simulink model "doc_interleaver"  (R2014a)
settings: Solver=ode45  SolverMode=SingleTasking  StartTime=0.0  StopTime=length(errors)  RelTol=1e-3
undefined symbols (not defined in the file or in its folder): gfprimfd
libraries: commblkcod2 x2, commblkintrlv2 x2, commrandsrc2 x1, commsink2 x1, simulink x1, dspsrcs4 x1
settings Model: Creator=The MathWorks Inc.
settings DataIOCC: SignalLoggingSaveFormat=ModelDataLogs  SaveOutput=off  SaveTime=off
settings OptimizationCC: BooleanDataType=off  InlineParams=on  ExpressionDepthLimit=2147483647
settings DebuggingCC: AlgebraicLoopMsg=error  SaveWithParameterizedLinksMsg=none  UnderspecifiedInitializationDetection=Classic  SignalResolutionControl=TryResolveAllWithWarning  SolverPrmCheckMsg=none  MultiTaskDSMMsg=warning  MultiTaskCondExecSysMsg=none  FcnCallInpInsideContextMsg=UseLocalSettings  StateNameClashWarn=warning  StrictBusMsg=None
settings HardwareCC: TargetUnknown=on
settings RTWCC: IncludeERTFirstTime=on
settings GRTTargetCC: CombineOutputUpdateFcns=off  GRTInterface=on

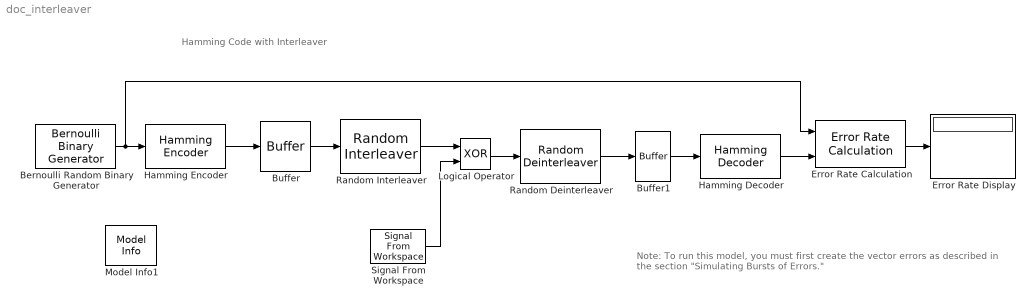
== system doc_interleaver ==
  note: Hamming Code with Interleaver
  note: Note: To run this model, you must first create the vector errors
      | as described in the section "Simulating Bursts of Errors."
  Bernoulli Random Binary Generator : commrandsrc2/Bernoulli Binary Generator  P=0.5  seed=435345  Ts=1  frameBased=on  sampPerFrame=4  orient=off  outDataType=double
  Buffer : Buffer  N=84  TreatMby1Signals=One channel
  Buffer1 : Buffer  N=7  TreatMby1Signals=One channel
  Error Rate Calculation : commsink2/Error Rate Calculation  N=(4/7)*84  st_delay=100  cp_mode=Entire frame  subframe=[]  PMode=Port  WsName=ErrorVec  RsMode2=off  stop=off  numErr=100  maxBits=1000
  Error Rate Display : Display
  Hamming Decoder : commblkcod2/Hamming Decoder  n=7  k=gfprimfd(3,'min')
  Hamming Encoder : commblkcod2/Hamming Encoder  n=7  k=gfprimfd(3,'min')
  Logical Operator : Logic  Operator=XOR
  Model Info1 : simulink/Model-Wide Utilities/Model Info  InitialBlockCM=None  BlockCM=None  Frame=on  DisplayStringWithTags=Info  HorizontalTextAlignment=Center  LeftAlignmentValue=0.5  SourceBlockDiagram=doc_interleaver  TagMaxNumber=20
  Random Deinterleaver : commblkintrlv2/Random Deinterleaver  N=84  seed=113
  Random Interleaver : commblkintrlv2/Random Interleaver  N=84  seed=113
  Signal From Workspace : dspsrcs4/Signal From Workspace  X=errors  Ts=4/7  nsamps=84  OutputAfterFinalValue=Setting to zero  ignoreOrWarnInputAndFrameLengths=off
  wires:
  Error Rate Calculation/1 -> Error Rate Display/1
  Hamming Decoder/1 -> Error Rate Calculation/2
  Hamming Encoder/1 -> Buffer/1
  Buffer/1 -> Random Interleaver/1
  Buffer1/1 -> Hamming Decoder/1
  Random Deinterleaver/1 -> Buffer1/1
  Random Interleaver/1 -> Logical Operator/1
  Logical Operator/1 -> Random Deinterleaver/1
  Bernoulli Random Binary Generator/1 -> Hamming Encoder/1, Error Rate Calculation/1
  Signal From Workspace/1 -> Logical Operator/2
